simulink model "Prescan_Carsim_0118_cs"  (R2019b)
settings: Solver=ode5  StartTime=0.0  StopTime=inf  FixedStep=1/1000  RelTol=1e-3
PreLoadFcn:
  | mbxruntime.callbacks.PreLoadFcn(bdroot);
PostLoadFcn:
  | mbxruntime.callbacks.PostLoadFcn(bdroot);
InitFcn:
  | mbxruntime.callbacks.InitFcn(bdroot);
  | Initialization_Func;
  | 
  | % load the InputBus data.
  | load osqpcecInputBus.mat;
StartFcn:
  | mbxruntime.callbacks.StartFcn(bdroot);
  | current_sys=gcs;
  | speedblock=Simulink.findBlocks(current_sys,'Name','speed_kmh_Gain');
  | h1=add_exec_event_listener(speedblock,'PostOutputs',@SpeedVisulization);
  | outblock=Simulink.findBlocks(current_sys,'Name','trajectorycurveoutput_Gain');
  | CurveTrajectoryListenerHandle=add_exec_event_listener(outblock,'PostOutputs',@TrajectoryCurve_CallBack);
  | lanedatablock=Simulink.findBlocks(current_sys,'Name','LaneData_Gain');
  | CurveLaneListenerHandle=add_exec_event_listener(lanedatablock,'PostOutputs',@CurveLane_CallBack);
StopFcn:
  | mbxruntime.callbacks.StopFcn(bdroot);
model workspace: external: MAT-File .\Prescan_Carsim_0118_cs_hws.mat (data not in the file)
values from neighbouring files (symbols this model uses):
  g = 9.8    [Initialization_Func.m]
  InitialPlanningParameter = [0,0,1,0,2,2,2,40,60]'    [Initialization_Func.m]
  Kf = 20000    [Initialization_Func.m]
  Kr = 20000    [Initialization_Func.m]
  Lr = 1.644    [Initialization_Func.m]
  M = 1275    [Initialization_Func.m]
  nG = 24    [Initialization_Func.m]
  V = 60/3.6    (= 16.6666666667)    [Initialization_Func.m]
  VehicleBaseLength = Lf+Lr    (= 2.66)    [Initialization_Func.m]
undefined symbols (not defined in the file or in its folder): AAx, AAy, AAz, AVx, AVy, AVz, Ax, Ay, Az, canChannel, DiscIntNeverNeededParam, InitialDPMPDF_Comfort, InitialDPMPDF_Efficiency, InitialDPMPDF_Safety, InitialPDF_DEM, mbxruntime, NormalisedTrajectoryIndicator_Pool, Parameter_Indicator_LookUpTable, Prescan_Carsim_1230_cs_0658e9ca1334a8be, Prescan_Carsim_1230_cs_08c5eb9a1bd7376a, Prescan_Carsim_1230_cs_6cfd759b89b9fc85, Prescan_Carsim_1230_cs_9435cc1cceb5050d, Prescan_Carsim_1230_cs_ac716d34d49f74ab, Prescan_Carsim_1230_cs_be02757d7f212dd5, Rational_Coefficient_Learning, SteeringWheel, TrajectoryIndicatorRange, Vx, Vy, Vz, WheelL0, WheelL1, WheelR0, WheelR1
libraries: canmsglib x11, dsparch4 x6, canlib x3, PreScanSimulinkLibrary x3, Solver_SF x1, autolibshared x1
(part 7 of 8)

== matlab function Prescan_Carsim_0118_cs/BMW_X5_SUV_1/DEM updating and Preference Estimation/UpdateDEM/Online DEM updating/Select the Next Trajectory  ==
  data: PriorPDF_DEM input; ExpectedNext_NormalisedTrajectoryIndicator output; PriorDPMPDF_Safety input; PriorDPMPDF_Comfort input; PriorDPMPDF_Efficiency input; ExpectedNext_QueryID output; NormalisedTrajectoryIndicator_Pool input; Evaluated_NormalisedTrajectoryIndicator input; LastPreference_NormalisedTrajectoryIndicator input; Rational_Coefficient_Learning input
function [ExpectedNext_NormalisedTrajectoryIndicator,ExpectedNext_QueryID] = fcn(PriorPDF_DEM,PriorDPMPDF_Safety,PriorDPMPDF_Comfort,PriorDPMPDF_Efficiency,NormalisedTrajectoryIndicator_Pool,Evaluated_NormalisedTrajectoryIndicator,LastPreference_NormalisedTrajectoryIndicator,Rational_Coefficient_Learning)

persistent PDF_WeightTable ID_PDFTable
if isempty(PDF_WeightTable)
    % Construct the WeightTable and the PDF_WeightTable by combining the
    % PDF_DEM and PDF_DPM
    Num_WeightDEM=size(PriorPDF_DEM,1);
    NumIndicator_DPM=[size(PriorDPMPDF_Safety,2)-1,size(PriorDPMPDF_Comfort,2)-1,size(PriorDPMPDF_Efficiency,2)-1];% zeros means only 1 indicator
    Num_WeightDPM=[size(PriorDPMPDF_Safety,1),size(PriorDPMPDF_Comfort,1),size(PriorDPMPDF_Efficiency,1)];
    PDF_WeightTable=zeros(prod(Num_WeightDPM)*Num_WeightDEM,sum(NumIndicator_DPM)+1);
    [X1,X2,X3,X4]=ndgrid((1:Num_WeightDPM(1))',(1:Num_WeightDPM(2))',(1:Num_WeightDPM(3))',(1: Num_WeightDEM)');
    ID_PDFTable=[X1(:),X2(:),X3(:),X4(:)];
%   PDF_WeightTable(:,1)=PriorDPMPDF_Safety(X1(:),1).*PriorDPMPDF_Comfort(X2(:),1).*PriorDPMPDF_Efficiency(X3(:),1).*PriorPDF_DEM(X4(:),1);
    PDF_WeightTable(:,2:end)=[(PriorDPMPDF_Safety(X1(:),2:end).*PriorPDF_DEM(X4(:),2)),(PriorDPMPDF_Comfort(X2(:),2:end).*PriorPDF_DEM(X4(:),3)),...
        (PriorDPMPDF_Efficiency(X3(:),2:end).*PriorPDF_DEM(X4(:),4))];% The last three column is the weight of S-C-E 
end
PDF_WeightTable(:,1)=PriorDPMPDF_Safety(ID_PDFTable(:,1),1).*PriorDPMPDF_Comfort(ID_PDFTable(:,2),1).*PriorDPMPDF_Efficiency(ID_PDFTable(:,3),1).*PriorPDF_DEM(ID_PDFTable(:,4),1);

%======= Select the Next Trajectory Used to Commare for the next loop
%=================
% 1, Calculate the expected information difference for each possible query
% This one needs further modification
Available_ID=setdiff((1:size(NormalisedTrajectoryIndicator_Pool,1)),unique(Evaluated_NormalisedTrajectoryIndicator));
Alternative_Query=NormalisedTrajectoryIndicator_Pool(Available_ID,:)-repmat(LastPreference_NormalisedTrajectoryIndicator,length(Available_ID),1);
Max_QueryID=Select_ExpectedInformationVolume(PriorPDF_DEM,PriorDPMPDF_Safety,PriorDPMPDF_Comfort,PriorDPMPDF_Efficiency,PDF_WeightTable,ID_PDFTable,Alternative_Query,Rational_Coefficient_Learning);
ExpectedNext_QueryID=Available_ID(Max_QueryID);
ExpectedNext_NormalisedTrajectoryIndicator=NormalisedTrajectoryIndicator_Pool(ExpectedNext_QueryID,:);
end

function max_queryID=Select_ExpectedInformationVolume(PriorPDF_DEM,PriorDPMPDF_Safety,PriorDPMPDF_Comfort,PriorDPMPDF_Efficiency,PDF_WeightTable,ID_PDFTable,Query_Pool,learning_rate_agent)
% calculate the expected difference between the prior and post probability
% density function for each query in the Query_Pool.
% PriorPDF_DEM: initial prob distribution of the DEM(S-C-E),Num_Weight_DEM*1;
% DEM_WeightSet : date array like Ndim*Num_discrete_theta
% Query_pool:data array like Ndim*Num_query
Num_Query=size(Query_Pool,1);
DEM_WeightSet=PriorPDF_DEM(:,2:end);
Num_WeightDEM=size(PriorPDF_DEM,1);

PDF_WeightTable(:,1)=PriorDPMPDF_Safety(ID_PDFTable(:,1),1).*PriorDPMPDF_Comfort(ID_PDFTable(:,2),1).*PriorDPMPDF_Efficiency(ID_PDFTable(:,3),1).*PriorPDF_DEM(ID_PDFTable(:,4),1);
LikeHood_1_WeightByQuery=LikeHood_Func(PDF_WeightTable(:,2:end),Query_Pool,1,learning_rate_agent);
Post_PDF=repmat(PDF_WeightTable(:,1),1,Num_Query).*LikeHood_1_WeightByQuery;

% the expected information difference of DEM
PostPDF_DEM=zeros(Num_WeightDEM,Num_Query);
for DEM_i=1:Num_WeightDEM
    PostPDF_DEM(DEM_i,:)=sum(Post_PDF(ID_PDFTable(:,4)==DEM_i,:),1);
end

[Post_PDFNorm,sum_post]=PDF_NormFunc(PostPDF_DEM,DEM_WeightSet);


Prob_Difference=abs(repmat(PriorPDF_DEM(:,1),1,Num_Query)-Post_PDFNorm);
[~,Sum_Prob_Difference]=PDF_NormFunc(Prob_Difference,DEM_WeightSet);
Expected_Information=Sum_Prob_Difference.*sum_post;
[~,max_queryID]=max(Expected_Information);
end

function [post_prob,sum_prob]=PDF_NormFunc(PDF,Weight_Set)
    % prob_distrib is a array of the post probability distribution. the row
    % number is the dicrete weight number,and the column number is the query/action.
    % each column is the post prob distribution of the query.
    % this function is to calculate the total prob in the considering
    % weight range to be 1
    % pdf_func: is a function handle.
   if size(PDF,1)==1
        post_prob=1;
        sum_prob=PDF;
    else
        uniqueweight=unique(Weight_Set(:,1));
        Interval_Weight=min(diff(uniqueweight));
        Ndim_ValidWeight=size(Weight_Set,2)-1;
        % considering the truth that the valid range of the independent variable
        if Ndim_ValidWeight==1
            sum_prob=sum(PDF(1:end-1))*Interval_Weight;
        else 
            pos_temp=sum(Weight_Set(:,1:Ndim_ValidWeight),2)<=1-Interval_Weight;
            sum_prob=sum(PDF(pos_temp,:))*Interval_Weight^Ndim_ValidWeight;
        end
        post_prob=PDF./repmat(sum_prob,size(PDF,1),1);
    end        
end

== matlab function Prescan_Carsim_0118_cs/BMW_X5_SUV_1/Trajectory Indicator Calculation/VehicleState_Buffer/VehicleInfo_StoreDuringCurve ==
  data: VehicleState_Var input; VehicleState_Curve output
function VehicleState_Curve= fcn(VehicleState_Var)
% Store the Vehicle State data during Curve Road
% #codegen
coder.extrinsic('warning');
%====Initialization of the Buffer
persistent Size_Limit VehicleState_Buffer Data_num Var_num
if isempty(Size_Limit)
    Var_num=17;
    Size_Limit=1000; % Change according to the sample rate and the time during the curve
    VehicleState_Buffer=zeros(Size_Limit,Var_num);
    Data_num=0;
end

if not(length(VehicleState_Var)==Var_num)
    warning('The Variable Number is not consistent!\n')
end
VehicleState_Curve=zeros(1000,17);

Data_num=Data_num+1;
if Data_num<=Size_Limit
    VehicleState_Buffer(Data_num,:)=VehicleState_Var;
else
    warning('The Size_Limit is short than the data length in the curve!\n')
end
VehicleState_Curve(1:Size_Limit,:)= VehicleState_Buffer;

== matlab function Prescan_Carsim_0118_cs/BMW_X5_SUV_1/trajectory planning/MATLAB Function1 ==
  data: PathPlan_FixedSize input; TargetPath_VariableSize output size=[1000 2]; PlanSpeed_FixedSize input; TargetSpeed_VariableSize output size=[1000 1]; DataLength_Plan input
function [TargetPath_VariableSize,TargetSpeed_VariableSize]  = fcn(PathPlan_FixedSize,PlanSpeed_FixedSize,DataLength_Plan)
TargetPath_VariableSize=PathPlan_FixedSize(1:DataLength_Plan,:);
TargetSpeed_VariableSize = PlanSpeed_FixedSize(1:DataLength_Plan,:);
end

== matlab function Prescan_Carsim_0118_cs/BMW_X5_SUV_1/trajectory planning/Generate Road Lane from Polyfit TLC calculation /TLC calculation and Lane Generation Road Lane  ==
  data: RoadLanePlan input size=[1000 4]; LateralOffset output; PolyRoadLane input; RoadLaneEnd_Rotation input; IntervalRoadSegment input; Width_Road input; Width_Vehicle input; Length_Vehicle input; Range input; YawRate input; Speed input; TLC_Left output; TLC_Right output
function [LateralOffset,TLC_Left,TLC_Right] = fcn(RoadLanePlan,PolyRoadLane,RoadLaneEnd_Rotation,IntervalRoadSegment,Width_Road,Width_Vehicle,Length_Vehicle,Range,YawRate,Speed)
% coder.extrinsic('fminlbfgs')
%,'getexitmessage','call_output_function','linesearch_simple','sectioningPhase','linesearch',...
%     'bracketingPhase','linesearch_simple','pickAlphaWithinInterval','gradient_function','updateQuasiNewtonMatrix_LBFGS');

LaneCenter_Local=0.5*[RoadLanePlan(:,1)+RoadLanePlan(:,3),RoadLanePlan(:,2)+RoadLanePlan(:,4)];
Range=150;
Order_polyfit=2;
% the path coordinates within the distance Before and after the current position are used to fit the path
options = struct('TolX',0.05,'TolFun',1e-2);

LaneCenter_Valid=LaneCenter_Local(LaneCenter_Local(:,1)<=Range & LaneCenter_Local(:,1)>=-1*Range,:);
PathPolyfit=polyfit(LaneCenter_Valid(:,1),LaneCenter_Valid(:,2),Order_polyfit);
Func_Pathfit=@(t) [t,polyval(PathPolyfit,t)];
OptFunc_Fit=@(t) (Func_Pathfit(t)-[0,0])*(Func_Pathfit(t)-[0,0])';
[~, fvalue]=fminbnd(OptFunc_Fit,-Range,Range,options);
if Func_Pathfit(0)<=0
    LateralOffset=sqrt(fvalue);
else
    LateralOffset=-1*sqrt(fvalue);
end


% Vehicle Wheel path Func
Func_roation_matrix=@(t)[cos(t),sin(t);-sin(t),cos(t)];% anti-clock rotation
ployrotationangle=deg2rad(45);
Rotationmatrix=Func_roation_matrix(ployrotationangle);
WheelOffset=0.5*[Length_Vehicle,Width_Vehicle];
R=sign(YawRate)*Speed./(abs(YawRate)+1e-6);% Positive means 
Func_VehCog_Local = @(t) [abs(R)*sin(t),R*(1-cos(t))];
Func_LeftWheel_LocalRot=@(t) (Func_VehCog_Local(t)+WheelOffset*Func_roation_matrix(t))*Rotationmatrix;
Func_RightWheel_LocalRot=@(t) (Func_VehCog_Local(t)-WheelOffset*Func_roation_matrix(t))*Rotationmatrix;
% Polyfit Lane 
LeftLanePolyfitRot=PolyRoadLane(:,2)';
Func_LaneLeft_LocalRot=@(t) [t,polyval(LeftLanePolyfitRot,t)];
RightLanePolyfitRot=PolyRoadLane(:,1)';
Func_LaneRight_LocalRot=@(t) [t,polyval(RightLanePolyfitRot,t)];

threshold_criteria=5e-2;
% options = struct('GradObj','off','Display','off','LargeScale','off','HessUpdate','bfgs','InitialHessType','identity','GoalsExactAchieve',1,'GradConstr',false,'TolFun',1e-2);
Optleftwheel=@(t) (Func_LeftWheel_LocalRot(t(1))-Func_LaneLeft_LocalRot(t(2)))*(Func_LeftWheel_LocalRot(t(1))-Func_LaneLeft_LocalRot(t(2)))';
[solutionleft, fvalue] = fminsearch(Optleftwheel,[0.03,20]);
solution_local=Func_LeftWheel_LocalRot(solutionleft(1))*Rotationmatrix';% coordination
if solution_local(1)>=0 && solution_local(1)<=Range && fvalue<threshold_criteria
    TLC_Left=R*solutionleft(1)/Speed+eps;
else
    TLC_Left=nan;
end

Optrightwheel=@(t) (Func_RightWheel_LocalRot(t(1))-Func_LaneRight_LocalRot(t(2)))*(Func_RightWheel_LocalRot(t(1))-Func_LaneRight_LocalRot(t(2)))';
[solutionright, fvalue] = fminsearch(Optrightwheel,[0.03,20]);
solution_local=Func_RightWheel_LocalRot(solutionright(1))*Rotationmatrix';% coordination
if solution_local(1)>=0 && solution_local(1)<=Range && fvalue<threshold_criteria
    TLC_Right=R*solutionright(1)/Speed+eps;
else
    TLC_Right=nan;
end

% Generate Road
LeftLanePoly=PolyRoadLane(:,2)';
rightlaneend_rotation=RoadLaneEnd_Rotation(3:4);
% Intergrate to find the sample road points with intervalsegment 
x_delta=linspace(0,rightlaneend_rotation(1),800);
y_fitvalue=polyval(LeftLanePoly,x_delta);
diff_length=sqrt(diff(x_delta).^2+diff(y_fitvalue).^2);
length_cumsum=[0,cumsum(diff_length)];
x_int4=0:IntervalRoadSegment:length_cumsum(end);
idx=zeros(1,length(x_int4));
for i=1:length(x_int4)
    idx(i)=find(length_cumsum>=x_int4(i),1);
end
rightlaneIntervalfited_rotation=[x_delta(idx)',y_fitvalue(idx)'];
RightLane_Plan=rightlaneIntervalfited_rotation*Rotationmatrix';
LeftLane_Plan=Made_VirtualLane(RightLane_Plan,1,Width_Road);
RoadLane_Plan=[LeftLane_Plan,RightLane_Plan];
%}

end

% Local Function
function [Lane_Virtual]=Made_VirtualLane(BaseLane,Flag_RightBase,Width_Road)
% made the virtual lane based on the baselane with a fixed road width
% 3.75m.
% BaseLane: a array like Num_roadpoint*2,the first column is the X
% coordinates while the other column is the Y coordinates.
% Flag_Right:a logical variable, if 1, it shows the baselane is the right
% one, if 0, the baselane is the left one.
% Lane_Virtual=zeros(1000,2);% a large data array to fix the size of the output.
Vec_BaseLane=zeros(size(BaseLane,1),2);
Vec_BaseLane(1:end-1,1)=BaseLane(2:end,1)-BaseLane(1:end-1,1);
Vec_BaseLane(end,1)=Vec_BaseLane(end-1,1);
Vec_BaseLane(1:end-1,2)=BaseLane(2:end,2)-BaseLane(1:end-1,2);
Vec_BaseLane(end,2)=Vec_BaseLane(end-1,2);
VecLength_BaseLane=sqrt(Vec_BaseLane(:,1).^2+Vec_BaseLane(:,2).^2);
Vec_BaseLane_unit=[Vec_BaseLane(:,1)./VecLength_BaseLane,Vec_BaseLane(:,2)./VecLength_BaseLane];
if Flag_RightBase==1
    Rotation_Transformation=[0,-1;1,0];
else
    Rotation_Transformation=[0,1;-1,0];
end
Vec_VirtualToBase=Rotation_Transformation*Vec_BaseLane_unit';% 2*N
Lane_Virtual=BaseLane+Width_Road*Vec_VirtualToBase';

end

function [x,fval,exitflag,output,grad]=fminlbfgs(funfcn,x_init,optim)
%FMINLBFGS finds a local minimum of a function of several variables. 
%   This optimizer is developed for image registration methods with large 
%	amounts of unknown variables.
%
%   Optimization methods supported:
%	- Quasi Newton Broyden letcher oldfarb hanno (BFGS)  
%   - Limited memory BFGS (L-BFGS)
%   - Steepest Gradient Descent optimization.
%   
%   [X,FVAL,EXITFLAG,OUTPUT,GRAD] = FMINLBFGS(FUN,X0,OPTIONS) 
%
%   Inputs,
%		FUN: Function handle or string which is minimized, returning an
%				error value and optional the error gradient. 
%		X0: Initial values of unknowns can be a scalar, vector or matrix
%	 (optional)
%		OPTIONS: Structure with optimizer options, made by a struct or
%				optimset. (optimset doesnot support all input options)
%
%   Outputs,
%		X : The found location (values) which minimize the function.
%		FVAL : The minimum found
%		EXITFLAG : Gives value, which explain why the minimizer stopt
%		OUTPUT : Structure with all important ouput values and parameters
%		GRAD : The gradient at this location 
%
%   Extended description of input/ouput variables 
%   OPTIONS,
%		OPTIONS.GoalsExactAchieve : If set to 0, a line search method is
%               used which uses a few function calls to do a good line
%               search. When set to 1 a normal line search method with Wolfe 
%				conditions is used (default).
%		OPTIONS.GradConstr, Set this variable to true if gradient calls are
%				cpu-expensive (default). If false more gradient calls are 
%				used and less function calls.
%	    OPTIONS.HessUpdate : If set to 'bfgs', Broyden letcher oldfarb hanno 
%				optimization is used (default), when the number of unknowns is 
%				larger then 3000 the function will switch to Limited memory BFGS, 
%				or if you set it to 'lbfgs'. When set to 'steepdesc', steepest 
%				decent optimization is used.
%		OPTIONS.StoreN : Number of itterations used to approximate the Hessian,
%			 	in L-BFGS, 20 is default. A lower value may work better with
%				non smooth functions, because than the Hessian is only valid for
%				a specific position. A higher value is recommend with quadratic equations. 
%		OPTIONS.GradObj : Set to 'on' if gradient available otherwise finited difference
%				is used.
%     	OPTIONS.Display : Level of display. 'off' displays no output; 'plot' displays
%				all linesearch results in figures. 'iter' displays output at  each 
%               iteration; 'final' displays just the final output; 'notify' 
%				displays output only if the function does not converge; 
%	    OPTIONS.TolX : Termination tolerance on x, default 1e-6.
%	    OPTIONS.TolFun : Termination tolerance on the function value, default 1e-6.
%		OPTIONS.MaxIter : Maximum number of iterations allowed, default 400.
% 		OPTIONS.MaxFunEvals : Maximum number of function evaluations allowed, 
%				default 100 times the amount of unknowns.
%		OPTIONS.DiffMaxChange : Maximum stepsize used for finite difference gradients.
%		OPTIONS.DiffMinChange : Minimum stepsize used for finite difference gradients.
%		OPTIONS.OutputFcn : User-defined function that an optimization function calls
%				at each iteration.
%		OPTIONS.rho : Wolfe condition on gradient (c1 on wikipedia), default 0.01.
%		OPTIONS.sigma : Wolfe condition on gradient (c2 on wikipedia), default 0.9. 
%		OPTIONS.tau1 : Bracket expansion if stepsize becomes larger, default 3.
%		OPTIONS.tau2 : Left bracket reduction used in section phase,
%		default 0.1.
%		OPTIONS.tau3 : Right bracket reduction used in section phase, default 0.5.
%   FUN,
%		The speed of this optimizer can be improved by also providing
%   	the gradient at X. Write the FUN function as follows
%   	function [f,g]=FUN(X)
%       	f , value calculation at X;
%   	if ( nargout > 1 )
%       	g , gradient calculation at X;
%   	end
%	EXITFLAG,
%		Possible values of EXITFLAG, and the corresponding exit conditions
%		are
%  		1, 'Change in the objective function value was less than the specified tolerance TolFun.';
%  		2, 'Change in x was smaller than the specified tolerance TolX.'; 
%  		3, 'Magnitude of gradient smaller than the specified tolerance';
%  		4, 'Boundary fminimum reached.';
%  		0, 'Number of iterations exceeded options.MaxIter or number of function evaluations exceeded options.FunEvals.';
%  		-1, 'Algorithm was terminated by the output function.';
%  		-2, 'Line search cannot find an acceptable point along the current search';
%
%   Examples
%       options = optimset('GradObj','on');
%       X = fminlbfgs(@myfun,2,options)
%
%   	% where myfun is a MATLAB function such as:
%       function [f,g] = myfun(x)
%       f = sin(x) + 3;
%	    if ( nargout > 1 ), g = cos(x); end
%
%   See also OPTIMSET, FMINSEARCH, FMINBND, FMINCON, FMINUNC, @, INLINE.
%
%   Function is written by D.Kroon University of Twente (Updated Nov. 2010)

% Read Optimalisation Parameters
defaultopt = struct('Display','final','HessUpdate','bfgs','GoalsExactAchieve',1,'GradConstr',true,  ...
			'TolX',1e-6,'TolFun',1e-6,'GradObj','off','MaxIter',400,'MaxFunEvals',100*numel(x_init)-1,  ...
			'DiffMaxChange',1e-1,'DiffMinChange',1e-8,'OutputFcn',[], ...
			'rho',0.0100,'sigma',0.900,'tau1',3,'tau2', 0.1, 'tau3', 0.5,'StoreN',20);

if (~exist('optim','var')) 
    optim=defaultopt;
else
    f = fieldnames(defaultopt);
    for i=1:length(f),
        if (~isfield(optim,f{i})||(isempty(optim.(f{i})))), optim.(f{i})=defaultopt.(f{i}); end
    end
end
    
% Initialize the data structure
data.fval=0;
data.gradient=0;
data.fOld=[]; 
data.xsizes=size(x_init);
data.numberOfVariables = numel(x_init);
data.xInitial = x_init(:);
data.alpha=1;
data.xOld=data.xInitial; 
data.iteration=0;
data.funcCount=0;
data.gradCount=0;
data.exitflag=[];
data.nStored=0;
data.timeTotal=tic;
data.timeExtern=0;
% Switch to L-BFGS in case of more than 3000 unknown variables
if(optim.HessUpdate(1)=='b') 
    if(data.numberOfVariables<3000), 
        optim.HessUpdate='bfgs';
    else
        optim.HessUpdate='lbfgs';
    end
end

if(optim.HessUpdate(1)=='l')
    succes=false;
    while(~succes)
        try
            data.deltaX=zeros(data.numberOfVariables,optim.StoreN);
            data.deltaG=zeros(data.numberOfVariables,optim.StoreN);
            data.saveD=zeros(data.numberOfVariables,optim.StoreN);
            succes=true;
        catch ME
            warning('fminlbfgs:memory','Decreasing StoreN value because out of memory');
            succes=false;
            data.deltaX=[]; data.deltaG=[]; data.saveD=[];
            optim.StoreN=optim.StoreN-1;
            if(optim.StoreN<1)
                rethrow(ME);
            end
        end
    end
end

exitflag=[];

% Display column headers
if(strcmp(optim.Display,'iter'))
    disp('     Iteration  Func-count   Grad-count         f(x)         Step-size');
end

% Calculate the initial error and gradient
data.initialStepLength=1;
[data,fval,grad]=gradient_function(data.xInitial,funfcn, data, optim);
data.gradient=grad;
data.dir = -data.gradient;
data.fInitial = fval;
data.fPrimeInitial= data.gradient'*data.dir(:);
data.fOld=data.fInitial;
data.xOld=data.xInitial;
data.gOld=data.gradient;
    

gNorm = norm(data.gradient,Inf);  % Norm of gradient
data.initialStepLength = min(1/gNorm,5); 

% Show the current iteration
if(strcmp(optim.Display,'iter'))
        s=sprintf('     %5.0f       %5.0f       %5.0f       %13.6g    ',data.iteration,data.funcCount,data.gradCount,data.fInitial); disp(s);
end
  
% Hessian intialization
if(optim.HessUpdate(1)=='b')
	data.Hessian=eye(data.numberOfVariables);
end

% Call output function
if(call_output_function(data,optim,'init')), exitflag=-1; end
    
% Start Minimizing
while(true)
    % Update number of itterations
    data.iteration=data.iteration+1; 

    % Set current lineSearch parameters
    data.TolFunLnS = eps(max(1,abs(data.fInitial )));
    data.fminimum = data.fInitial - 1e16*(1+abs(data.fInitial));
    
	% Make arrays to store linesearch results
    data.storefx=[]; data.storepx=[]; data.storex=[]; data.storegx=[];

    % If option display plot, than start new figure
    if(optim.Display(1)=='p'), figure, hold on; end
		
    % Find a good step size in the direction of the gradient: Linesearch
    if(optim.GoalsExactAchieve==1)
		data=linesearch(funfcn, data,optim);
    else
        data=linesearch_simple(funfcn, data, optim);
    end
	
	% Make linesearch plot
	if(optim.Display(1)=='p'); 
		plot(data.storex,data.storefx,'r*');
		plot(data.storex,data.storefx,'b');
		
		alpha_test= linspace(min(data.storex(:))/3, max(data.storex(:))*1.3, 10);
		falpha_test=zeros(1,length(alpha_test));
        for i=1:length(alpha_test)
			[data,falpha_test(i)]=gradient_function(data.xInitial(:)+alpha_test(i)*data.dir(:),funfcn, data, optim);
        end    
		plot(alpha_test,falpha_test,'g');
        plot(data.alpha,data.f_alpha,'go','MarkerSize',8);
	end
	
    % Check if exitflag is set
    if(~isempty(data.exitflag))
        exitflag=data.exitflag;
        data.xInitial=data.xOld; 
        data.fInitial=data.fOld;
        data.gradient=data.gOld;
        break 
    end
    
    % Update x with the alpha step
    data.xInitial = data.xInitial + data.alpha*data.dir;
    
    % Set the current error and gradient
    data.fInitial =  data.f_alpha;
	data.gradient = data.grad;
    
    % Set initial steplength to 1
    data.initialStepLength = 1;
    
    
    gNorm = norm(data.gradient,Inf);  % Norm of gradient
    
    % Set exit flags 
    if(gNorm <optim.TolFun), exitflag=1; end
    if(max(abs(data.xOld-data.xInitial)) <optim.TolX), exitflag=2; end
    if(data.iteration>=optim.MaxIter), exitflag=0; end
    
    % Check if exitflag is set
    if(~isempty(exitflag)), break, end

    % Update the inverse Hessian matrix
    if(optim.HessUpdate(1)~='s')
        % Do the Quasi-Neton Hessian update.
        data = updateQuasiNewtonMatrix_LBFGS(data,optim);
    else
        data.dir = -data.gradient;
    end
  
    % Derivative of direction
    data.fPrimeInitial= data.gradient'*data.dir(:);

    % Call output function
    if(call_output_function(data,optim,'iter')), exitflag=-1; end
    
    % Show the current iteration
    if(strcmp(optim.Display(1),'i')||strcmp(optim.Display(1),'p'))
        s=sprintf('     %5.0f       %5.0f       %5.0f       %13.6g   %13.6g',data.iteration,data.funcCount,data.gradCount,data.fInitial,data.alpha); disp(s);
    end
    
    % Keep the variables for next iteration
    data.fOld=data.fInitial;
    data.xOld=data.xInitial;
    data.gOld=data.gradient;
end
% Set output parameters
fval=data.fInitial;
grad=data.gradient;
x = data.xInitial;

% Reshape x to original shape
x=reshape(x,data.xsizes);

% Call output function
if(call_output_function(data,optim,'done')), exitflag=-1; end

% Make exist output structure
if(optim.HessUpdate(1)=='b'), output.algorithm='Broyden letcher oldfarb hanno (BFGS)';
elseif(optim.HessUpdate(1)=='l'), output.algorithm='limited memory BFGS (L-BFGS)';
else output.algorithm='Steepest Gradient Descent'; 
end
output.message=getexitmessage(exitflag);
output.iteration = data.iteration;
output.funccount = data.funcCount;
output.fval = data.fInitial;
output.stepsize = data.alpha;
output.directionalderivative = data.fPrimeInitial;
output.gradient = reshape(data.gradient, data.xsizes);
output.searchdirection = data.dir;
output.timeTotal=toc(data.timeTotal);    
output.timeExtern=data.timeExtern;
oupput.timeIntern=output.timeTotal-output.timeExtern;
% Display final results
if(~strcmp(optim.Display,'off'))
    disp('    Optimizer Results')
    disp(['        Algorithm Used: ' output.algorithm]);
    disp(['        Exit message : ' output.message]);
    disp(['        iterations : '  int2str(data.iteration)]);
    disp(['        Function Count : ' int2str(data.funcCount)]);
    disp(['        Minimum found : ' num2str(fval)]);
    disp(['        Intern Time : ' num2str(oupput.timeIntern) ' seconds']);
    disp(['        Total Time : ' num2str(output.timeTotal) ' seconds']);
end
end
function message=getexitmessage(exitflag)
    switch(exitflag)
        case 1, message='Change in the objective function value was less than the specified tolerance TolFun.';
        case 2, message='Change in x was smaller than the specified tolerance TolX.'; 
        case 3, message='Magnitude of gradient smaller than the specified tolerance';
        case 4, message='Boundary fminimum reached.';
        case 0, message='Number of iterations exceeded options.MaxIter or number of function evaluations exceeded options.FunEvals.';
        case -1, message='Algorithm was terminated by the output function.';
        case -2, message='Line search cannot find an acceptable point along the current search';
        otherwise, message='Undefined exit code';
    end
end
    
function stopt=call_output_function(data,optim,where)
stopt=false;
if(~isempty(optim.OutputFcn))
    output.iteration = data.iteration;
    output.funccount = data.funcCount;
    output.fval = data.fInitial;
    output.stepsize = data.alpha;
    output.directionalderivative = data.fPrimeInitial;
    output.gradient = reshape(data.gradient, data.xsizes);
    output.searchdirection = data.dir;
    stopt=feval(optim.OutputFcn,reshape(data.xInitial,data.xsizes),output,where); 
end
end      
	
function data=linesearch_simple(funfcn, data, optim)
% Find a bracket of acceptable points
data = bracketingPhase_simple(funfcn, data, optim);

if (data.bracket_exitflag  == 2)
  % BracketingPhase found a bracket containing acceptable points; 
  % now find acceptable point within bracket
  data = sectioningPhase_simple(funfcn, data, optim);
  data.exitflag = data.section_exitflag; 
else
  % Already acceptable point found or MaxFunEvals reached
  data.exitflag = data.bracket_exitflag; 
end
end
function data = bracketingPhase_simple(funfcn, data,optim)
% Number of itterations
itw=0; 

% Point with smaller value, initial
data.beta=0; 
data.f_beta=data.fInitial; 
data.fPrime_beta=data.fPrimeInitial;

% Initial step is equal to alpha of previous step.
alpha = data.initialStepLength;

% Going up hill
hill=false;

% Search for brackets
while(true)
    % Calculate the error registration gradient
    if(optim.GradConstr)
        [data,f_alpha]=gradient_function(data.xInitial(:)+alpha*data.dir(:),funfcn, data, optim);
        fPrime_alpha=nan;
        grad=nan;
    else
        [data,f_alpha, grad]=gradient_function(data.xInitial(:)+alpha*data.dir(:),funfcn, data,optim);
        fPrime_alpha = grad'*data.dir(:);
    end
    
	% Store values linesearch
	data.storefx=[data.storefx f_alpha]; 
    data.storepx=[data.storepx fPrime_alpha]; 
	data.storex=[data.storex alpha]; 
	data.storegx=[data.storegx grad(:)];
    
    % Update step value
    if(data.f_beta<f_alpha), 
        % Go to smaller stepsize
        alpha=alpha*optim.tau3;
        
        % Set hill variable
        hill=true;
    else
        % Save current minium point
        data.beta=alpha; data.f_beta=f_alpha; data.fPrime_beta=fPrime_alpha; data.grad=grad;
        if(~hill)
            alpha=alpha*optim.tau1;  
        end
    end
                        
    % Update number of loop iterations
    itw=itw+1; 
		
    if(itw>(log(optim.TolFun)/log(optim.tau3))),
      % No new optium found, linesearch failed.
      data.bracket_exitflag=-2; break; 
    end
    
    if(data.beta>0&&hill)
            % Get the brackets around minimum point
            % Pick bracket A from stored trials
            [t,i]=sort(data.storex,'ascend');
            storefx=data.storefx(i);storepx=data.storepx(i); storex=data.storex(i);
            [t,i]=find(storex>data.beta,1);
            if(isempty(i)), [t,i]=find(storex==data.beta,1); end
            alpha=storex(i); f_alpha=storefx(i); fPrime_alpha=storepx(i);
            
            % Pick bracket B from stored trials
            [t,i]=sort(data.storex,'descend');
            storefx=data.storefx(i);storepx=data.storepx(i); storex=data.storex(i);
            [t,i]=find(storex<data.beta,1);
            if(isempty(i)), [t,i]=find(storex==data.beta,1); end
            beta=storex(i); f_beta=storefx(i); fPrime_beta=storepx(i);
            
            % Calculate derivatives if not already calculated
            if(optim.GradConstr)
                gstep=data.initialStepLength/1e6; 
                if(gstep>optim.DiffMaxChange), gstep=optim.DiffMaxChange; end
                if(gstep<optim.DiffMinChange), gstep=optim.DiffMinChange; end
                [data,f_alpha2]=gradient_function(data.xInitial(:)+(alpha+gstep)*data.dir(:),funfcn, data, optim);
                [data,f_beta2]=gradient_function(data.xInitial(:)+(beta+gstep)*data.dir(:),funfcn, data, optim);
                fPrime_alpha=(f_alpha2-f_alpha)/gstep;
                fPrime_beta=(f_beta2-f_beta)/gstep;
            end

            % Set the brackets A and B
            data.a=alpha; data.f_a=f_alpha; data.fPrime_a=fPrime_alpha;
            data.b=beta; data.f_b=f_beta; data.fPrime_b=fPrime_beta;
  
            % Finished bracketing phase
            data.bracket_exitflag  = 2; return
    end

	% Reached max function evaluations
	if(data.funcCount>=optim.MaxFunEvals), data.bracket_exitflag=0; return; end
end
end   

function data = sectioningPhase_simple(funfcn, data, optim)
% Get the brackets
brcktEndpntA=data.a; brcktEndpntB=data.b;

% Calculate minimum between brackets
[alpha,f_alpha_estimated] = pickAlphaWithinInterval(brcktEndpntA,brcktEndpntB,data.a,data.b,data.f_a,data.fPrime_a,data.f_b,data.fPrime_b,optim);  
if(isfield(data,'beta')&&(data.f_beta<f_alpha_estimated)), alpha=data.beta; end


[t,i]=find(data.storex==alpha,1);
if((~isempty(i))&&(~isnan(data.storegx(i))))
    f_alpha=data.storefx(i); grad=data.storegx(:,i);
else
    % Calculate the error and gradient for the next minimizer itteration
    [data,f_alpha, grad]=gradient_function(data.xInitial(:)+alpha*data.dir(:),funfcn, data,optim);
    if(isfield(data,'beta')&&(data.f_beta<f_alpha)), 
        alpha=data.beta; 
        if((~isempty(i))&&(~isnan(data.storegx(i))))
            f_alpha=data.storefx(i); grad=data.storegx(:,i);
        else
            [data,f_alpha, grad]=gradient_function(data.xInitial(:)+alpha*data.dir(:),funfcn, data,optim);
        end
    end
end

% Store values linesearch
data.storefx=[data.storefx f_alpha]; data.storex=[data.storex alpha];

fPrime_alpha = grad'*data.dir(:);
data.alpha=alpha; 
data.fPrime_alpha= fPrime_alpha; 
data.f_alpha= f_alpha;
data.grad=grad;

% Set the exit flag to succes   
data.section_exitflag=[];
end

function data=linesearch(funfcn, data, optim)

% Find a bracket of acceptable points
data = bracketingPhase(funfcn, data,optim);

if (data.bracket_exitflag  == 2)
  % BracketingPhase found a bracket containing acceptable points; 
  % now find acceptable point within bracket
  data = sectioningPhase(funfcn, data, optim);
  data.exitflag = data.section_exitflag; 
else
  % Already acceptable point found or MaxFunEvals reached
  data.exitflag = data.bracket_exitflag; 
end
end
function data = sectioningPhase(funfcn, data, optim)
%
% sectioningPhase finds an acceptable point alpha within a given bracket [a,b] 
% containing acceptable points. Notice that funcCount counts the total number of 
% function evaluations including those of the bracketing phase. 

while(true)
    
    % Pick alpha in reduced bracket
    brcktEndpntA = data.a + min(optim.tau2,optim.sigma)*(data.b - data.a); 
    brcktEndpntB = data.b - optim.tau3*(data.b - data.a);
    
    % Find global minimizer in bracket [brcktEndpntA,brcktEndpntB] of 3rd-degree 
    % polynomial that interpolates f() and f'() at "a" and at "b".
    alpha = pickAlphaWithinInterval(brcktEndpntA,brcktEndpntB,data.a,data.b,data.f_a,data.fPrime_a,data.f_b,data.fPrime_b,optim);  

    % No acceptable point could be found
    if (abs( (alpha - data.a)*data.fPrime_a ) <= data.TolFunLnS), data.section_exitflag = -2; return; end
    
    % Calculate value (and gradient if no extra time cost) of current alpha
    if(~optim.GradConstr)
        [data,f_alpha, grad]=gradient_function(data.xInitial(:)+alpha*data.dir(:),funfcn, data, optim);
        fPrime_alpha = grad'*data.dir(:);
    else
        gstep=data.initialStepLength/1e6; 
        if(gstep>optim.DiffMaxChange), gstep=optim.DiffMaxChange; end
        if(gstep<optim.DiffMinChange), gstep=optim.DiffMinChange; end
        [data,f_alpha]=gradient_function(data.xInitial(:)+alpha*data.dir(:),funfcn, data,optim);
        [data,f_alpha2]=gradient_function(data.xInitial(:)+(alpha+gstep)*data.dir(:),funfcn, data, optim);
        fPrime_alpha=(f_alpha2-f_alpha)/gstep;
    end

	% Store values linesearch 
	data.storefx=[data.storefx f_alpha]; data.storex=[data.storex alpha]; 
	
    % Store current bracket position of A
    aPrev = data.a; 
    f_aPrev = data.f_a; 
    fPrime_aPrev = data.fPrime_a; 

    % Update the current brackets
    if ((f_alpha > data.fInitial + alpha*optim.rho*data.fPrimeInitial) || (f_alpha >= data.f_a))
        % Update bracket B to current alpha
        data.b = alpha; data.f_b = f_alpha; data.fPrime_b = fPrime_alpha;
    else
        % Wolfe conditions, if true then acceptable point found 
        if (abs(fPrime_alpha) <= -optim.sigma*data.fPrimeInitial), 
            if(optim.GradConstr)
                % Gradient was not yet calculated because of time costs
                [data,f_alpha, grad]=gradient_function(data.xInitial(:)+alpha*data.dir(:),funfcn, data, optim);
                fPrime_alpha = grad'*data.dir(:);
            end
            % Store the found alpha values
            data.alpha=alpha; data.fPrime_alpha= fPrime_alpha; data.f_alpha= f_alpha;
            data.grad=grad;
            data.section_exitflag = []; return, 
        end
        
        % Update bracket A
        data.a = alpha; data.f_a = f_alpha;  data.fPrime_a = fPrime_alpha;
        
        if (data.b - data.a)*fPrime_alpha >= 0
            % B becomes old bracket A;
            data.b = aPrev; data.f_b = f_aPrev;  data.fPrime_b = fPrime_aPrev;
        end
    end
    
    % No acceptable point could be found
    if (abs(data.b-data.a) < eps), data.section_exitflag = -2; return, end

    % maxFunEvals reached
    if(data.funcCount >optim.MaxFunEvals), data.section_exitflag = -1; return, end
end
end
function data = bracketingPhase(funfcn, data, optim)
% bracketingPhase finds a bracket [a,b] that contains acceptable points; a bracket 
% is the same as a closed interval, except that a > b is allowed.
%
% The outputs f_a and fPrime_a are the values of the function and the derivative 
% evaluated at the bracket endpoint 'a'. Similar notation applies to the endpoint 
% 'b'. 

% Parameters of bracket A
data.a = []; 
data.f_a = []; 
data.fPrime_a = []; 

% Parameters of bracket B
data.b = []; 
data.f_b = []; 
data.fPrime_b = [];

% First trial alpha is user-supplied
% f_alpha will contain f(alpha) for all trial points alpha
% fPrime_alpha will contain f'(alpha) for all trial points alpha
alpha = data.initialStepLength;
f_alpha = data.fInitial;              
fPrime_alpha = data.fPrimeInitial;    

% Set maximum value of alpha (determined by fminimum)
alphaMax = (data.fminimum - data.fInitial)/(optim.rho*data.fPrimeInitial); 
alphaPrev = 0;

while(true) 
  % Evaluate f(alpha) and f'(alpha)
  fPrev = f_alpha;
  fPrimePrev = fPrime_alpha;
  
  % Calculate value (and gradient if no extra time cost) of current alpha
  if(~optim.GradConstr)
      [data,f_alpha, grad]=gradient_function(data.xInitial(:)+alpha*data.dir(:),funfcn, data, optim);
      fPrime_alpha = grad'*data.dir(:);
  else
      gstep=data.initialStepLength/1e6;
      if(gstep>optim.DiffMaxChange), gstep=optim.DiffMaxChange; end
      if(gstep<optim.DiffMinChange), gstep=optim.DiffMinChange; end
      [data,f_alpha]=gradient_function(data.xInitial(:)+alpha*data.dir(:),funfcn, data, optim);
      [data,f_alpha2]=gradient_function(data.xInitial(:)+(alpha+gstep)*data.dir(:),funfcn, data, optim);
      fPrime_alpha=(f_alpha2-f_alpha)/gstep;
  end
  
  % Store values linesearch 
  data.storefx=[data.storefx f_alpha]; data.storex=[data.storex alpha]; 
	
  % Terminate if f < fminimum
  if (f_alpha <= data.fminimum), data.bracket_exitflag = 4; return; end
  
  % Bracket located - case 1 (Wolfe conditions)
  if (f_alpha > (data.fInitial + alpha*optim.rho*data.fPrimeInitial)) || (f_alpha >= fPrev)
    % Set the bracket values
    data.a = alphaPrev; data.f_a = fPrev;  data.fPrime_a = fPrimePrev;
    data.b = alpha; data.f_b = f_alpha;  data.fPrime_b = fPrime_alpha;
    % Finished bracketing phase
    data.bracket_exitflag  = 2; return 
  end

  % Acceptable steplength found
  if (abs(fPrime_alpha) <= -optim.sigma*data.fPrimeInitial), 
      if(optim.GradConstr)
          % Gradient was not yet calculated because of time costs
          [data,f_alpha, grad]=gradient_function(data.xInitial(:)+alpha*data.dir(:),funfcn, data, optim);
          fPrime_alpha = grad'*data.dir(:);
      end
      % Store the found alpha values
      data.alpha=alpha;
      data.fPrime_alpha= fPrime_alpha; data.f_alpha= f_alpha; data.grad=grad;
      % Finished bracketing phase, and no need to call sectioning phase
      data.bracket_exitflag = [];  return 
  end
  
  % Bracket located - case 2  
  if (fPrime_alpha >= 0)
    % Set the bracket values
    data.a = alpha; data.f_a = f_alpha;  data.fPrime_a = fPrime_alpha;
    data.b = alphaPrev; data.f_b = fPrev; data.fPrime_b = fPrimePrev;
    % Finished bracketing phase
    data.bracket_exitflag  = 2; return
  end
 
  % Update alpha
  if (2*alpha - alphaPrev < alphaMax )
      brcktEndpntA = 2*alpha-alphaPrev; 
      brcktEndpntB = min(alphaMax,alpha+optim.tau1*(alpha-alphaPrev));
      % Find global minimizer in bracket [brcktEndpntA,brcktEndpntB] of 3rd-degree polynomial 
      % that interpolates f() and f'() at alphaPrev and at alpha
      alphaNew = pickAlphaWithinInterval(brcktEndpntA,brcktEndpntB,alphaPrev,alpha,fPrev, ...
                                         fPrimePrev,f_alpha,fPrime_alpha,optim);
      alphaPrev = alpha;
      alpha = alphaNew;
  else
      alpha = alphaMax;
  end

  % maxFunEvals reached
  if(data.funcCount >optim.MaxFunEvals), data.bracket_exitflag = -1; return, end
end
end
function [alpha,f_alpha]= pickAlphaWithinInterval(brcktEndpntA,brcktEndpntB,alpha1,alpha2,f1,fPrime1,f2,fPrime2,optim)
% finds a global minimizer alpha within the bracket [brcktEndpntA,brcktEndpntB] of the cubic polynomial 
% that interpolates f() and f'() at alpha1 and alpha2. Here f(alpha1) = f1, f'(alpha1) = fPrime1, 
% f(alpha2) = f2, f'(alpha2) = fPrime2.

% determines the coefficients of the cubic polynomial with c(alpha1) = f1, 
% c'(alpha1) = fPrime1, c(alpha2) = f2, c'(alpha2) = fPrime2.
coeff = [(fPrime1+fPrime2)*(alpha2-alpha1)-2*(f2-f1) ...
    3*(f2-f1)-(2*fPrime1+fPrime2)*(alpha2-alpha1) (alpha2-alpha1)*fPrime1 f1];

% Convert bounds to the z-space
lowerBound = (brcktEndpntA - alpha1)/(alpha2 - alpha1);
upperBound = (brcktEndpntB - alpha1)/(alpha2 - alpha1);

% Swap if lowerbound is higher than the upperbound
if (lowerBound  > upperBound), t=upperBound; upperBound=lowerBound; lowerBound=t; end 

% Find minima and maxima from the roots of the derivative of the polynomial.
sPoints = roots([3*coeff(1) 2*coeff(2) coeff(3)]); 

% Remove imaginaire and points outside range

sPoints(imag(sPoints)~=0)=[]; 
sPoints(sPoints<lowerBound)=[]; sPoints(sPoints>upperBound)=[];

% Make vector with all possible solutions
sPoints=[lowerBound sPoints(:)' upperBound];

% Select the global minimum point
[f_alpha,index]=min(polyval(coeff,sPoints)); z=sPoints(index);

% Add the offset and scale back from [0..1] to the alpha domain
alpha = alpha1 + z*(alpha2 - alpha1);

% Show polynomial search
if(optim.Display(1)=='p'); 
    vPoints=polyval(coeff,sPoints);
    plot(sPoints*(alpha2 - alpha1)+alpha1,vPoints,'co');
    plot([sPoints(1) sPoints(end)]*(alpha2 - alpha1)+alpha1,[vPoints(1) vPoints(end)],'c*');
    xPoints=linspace(lowerBound/3, upperBound*1.3, 50);
    vPoints=polyval(coeff,xPoints);
    plot(xPoints*(alpha2 - alpha1)+alpha1,vPoints,'c');
end
end	

function [data,fval,grad]=gradient_function(x,funfcn, data, optim)
    % Call the error function for error (and gradient)
    if ( nargout <3 )
        timem=tic;   
        fval=funfcn(reshape(x,data.xsizes)); 
        data.timeExtern=data.timeExtern+toc(timem);
        data.funcCount=data.funcCount+1;
    else
        if(strcmp(optim.GradObj,'on'))
            timem=tic;    
            [fval, grad]=feval(funfcn,reshape(x,data.xsizes)); 
            data.timeExtern=data.timeExtern+toc(timem);
            data.funcCount=data.funcCount+1;
            data.gradCount=data.gradCount+1;
        else
            % Calculate gradient with forward difference if not provided by the function
            grad=zeros(length(x),1);
            fval=funfcn(reshape(x,data.xsizes));
            gstep=data.initialStepLength/1e6; 
            if(gstep>optim.DiffMaxChange), gstep=optim.DiffMaxChange; end
            if(gstep<optim.DiffMinChange), gstep=optim.DiffMinChange; end
            for i=1:length(x),
                x_temp=x; x_temp(i)=x_temp(i)+gstep;
                timem=tic;    
                [fval_g]=feval(funfcn,reshape(x_temp,data.xsizes)); data.funcCount=data.funcCount+1;
                data.timeExtern=data.timeExtern+toc(timem);
                grad(i)=(fval_g-fval)/gstep;
            end
        end
        grad=grad(:);
    end
end  
function data = updateQuasiNewtonMatrix_LBFGS(data,optim)
% updates the quasi-Newton matrix that approximates the inverse to the Hessian.
% Two methods are support BFGS and L-BFGS, in L-BFGS the hessian is not
% constructed or stored.
% Calculate position, and gradient diference between the
% itterations
deltaX=data.alpha* data.dir;
deltaG=data.gradient-data.gOld;
        
if ((deltaX'*deltaG) >= sqrt(eps)*max( eps,norm(deltaX)*norm(deltaG) ))

    if(optim.HessUpdate(1)=='b')
        % Default BFGS as described by Nocedal
        p_k = 1 / (deltaG'*deltaX);
        Vk = eye(data.numberOfVariables) - p_k*deltaG*deltaX';
        % Set Hessian
        data.Hessian = Vk'*data.Hessian *Vk + p_k * deltaX*deltaX';
        % Set new Direction
        data.dir = -data.Hessian*data.gradient;
    else
        % L-BFGS with scaling as described by Nocedal
       
        % Update a list with the history of deltaX and deltaG
        data.deltaX(:,2:optim.StoreN)=data.deltaX(:,1:optim.StoreN-1); data.deltaX(:,1)=deltaX;
        data.deltaG(:,2:optim.StoreN)=data.deltaG(:,1:optim.StoreN-1); data.deltaG(:,1)=deltaG;
    
        data.nStored=data.nStored+1; if(data.nStored>optim.StoreN), data.nStored=optim.StoreN; end

        % Initialize variables
        a=zeros(1,data.nStored);
        p=zeros(1,data.nStored);

        q = data.gradient;
        for i=1:data.nStored
            p(i)= 1 / (data.deltaG(:,i)'*data.deltaX(:,i));
            a(i) = p(i)* data.deltaX(:,i)' * q;
            q = q - a(i) * data.deltaG(:,i);
        end
        % Scaling of initial Hessian (identity matrix)
        p_k = data.deltaG(:,1)'*data.deltaX(:,1) / sum(data.deltaG(:,1).^2); 
        
        % Make r = - Hessian * gradient
        r = p_k * q;
        for i=data.nStored:-1:1,
            b = p(i) * data.deltaG(:,i)' * r;
            r = r + data.deltaX(:,i)*(a(i)-b);
        end
        
        % Set new direction
        data.dir = -r;
    end
end
end
